simulink model "Requirements_Table"  (R2022b)
settings: Solver=FixedStepAuto  StartTime=0.0  StopTime=10.0  FixedStep=1e-3  RelTol=1e-3  EnableMultiTasking=on
undefined symbols (not defined in the file): D0, D1, D10, D11, D12, D13, D2, D3, D4, D5, D6, D7, D8, D9, PTA0, PTA1, PTA2, PTB23, PTB9, PTC16, PTC17, PTC2, PTC3, PTC4, PTD0, PTD1, PTD2, PTD3
libraries: frdmk64flib x17
settings Model: ExtModeTrigDuration=5  Creator=sarahalabdulrazzak  LastModifiedBy=shaydarahmatyan
settings SolverCC: AlgebraicLoopSolver=TrustRegion
settings OptimizationCC: EnhancedBackFolding=on  PassReuseOutputArgsAs=Individual arguments  ZeroExternalMemoryAtStartup=off  ZeroInternalMemoryAtStartup=off  MaxStackSize=64  OptimizeBlockOrder=speed  DifferentSizesBufferReuse=on  OptimizationCustomize=off  EfficientTunableParamExpr=on
settings DebuggingCC: ParameterTunabilityLossMsg=error  UnconnectedInputMsg=warning  UnconnectedOutputMsg=warning  UnconnectedLineMsg=warning  SFMachineParentedDataDiag=warning
settings HardwareCC: ProdBitPerPointer=32  ProdBitPerSizeT=32  ProdBitPerPtrDiffT=32  ProdLargestAtomicInteger=Long  ProdLargestAtomicFloat=Double  ProdWordSize=32  ProdHWDeviceType=ARM Compatible->ARM Cortex
settings ModelReferenceCC: EnableRefExpFcnMdlSchedulingChecks=on
settings SFSimCC: MATLABDynamicMemAlloc=off
settings RTWCC: Description=Embedded Coder  SystemTargetFile=ert.tlc  HardwareBoard=NXP FRDM-K64F  TLCOptions="-aInlineSetEventsForThisBaseRateFcn=TLC_FALSE -aSuppressMultiTaskScheduler=TLC_FALSE  -aRateBasedStepFcn=0"  TemplateMakefile=ert_default_tmf  Toolchain=GNU Tools for ARM Embedded Processors
settings CodeAppCC: ForceParamTrailComments=on  IgnoreCustomStorageClasses=off  OperatorAnnotations=on  SimulinkDataObjDesc=on  SFDataObjDesc=on  InsertBlockDesc=on

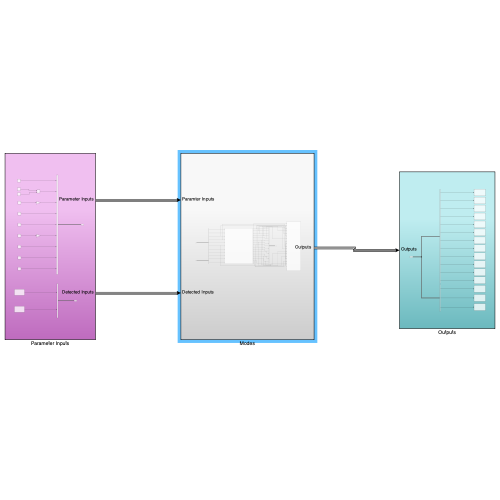
[thumbnail: Simulink's stored preview of the top-level diagram]
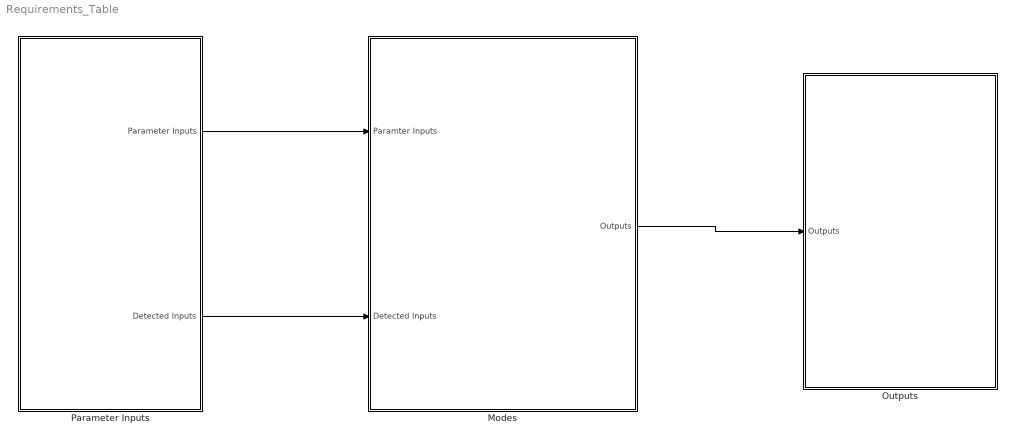
== system Requirements_Table ==
  Modes : Subsystem
  Outputs : Subsystem
  Parameter Inputs : Subsystem
  wires:
  Parameter Inputs/1(Parameter Inputs) -> Modes/1(Paramter Inputs)
  Parameter Inputs/2(Detected Inputs) -> Modes/2(Detected Inputs)
  Modes/1("Outputs ") -> Outputs/1("Outputs ")

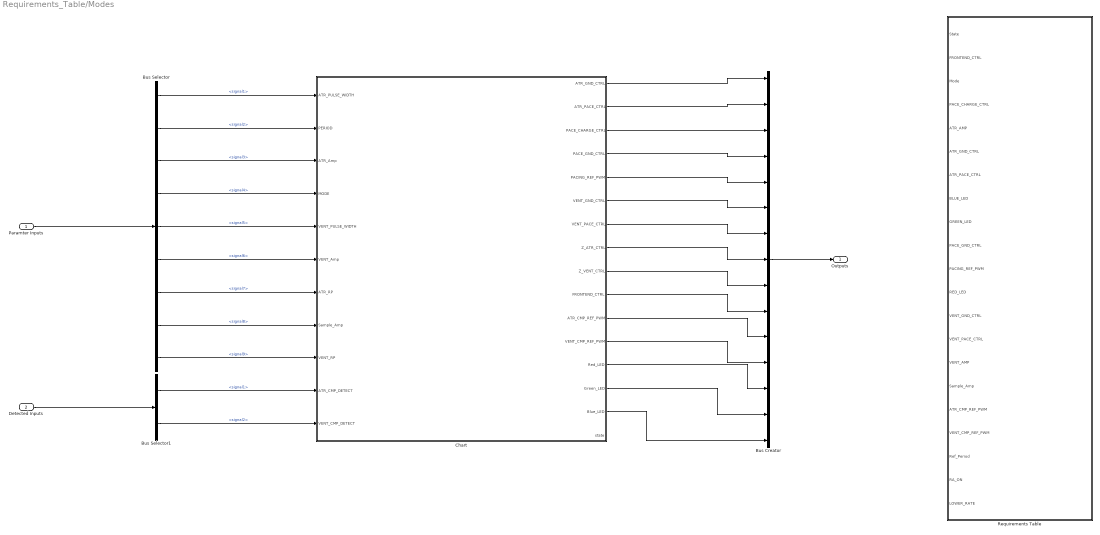
== system Requirements_Table/Modes ==
  Paramter Inputs : Inport
  Detected Inputs : Inport  Port=2
  Bus Creator : BusCreator  Inputs=15
  Bus Selector : BusSelector  OutputSignals=signal1,signal2,signal3,signal4,signal5,signal6,signal7,signal8,signal9
  Bus Selector1 : BusSelector  OutputSignals=signal1,signal2
  Chart : Stateflow chart  TreatAsAtomicUnit=on
  Requirements Table : Requirements Table  TreatAsAtomicUnit=on
  "Outputs " : Outport
  wires:
  Paramter Inputs/1 -> Bus Selector/1
  Detected Inputs/1 -> Bus Selector1/1
  Bus Selector/4 -> Chart/4(MODE)  "<signal4>"
  Bus Selector/5 -> Chart/5(VENT_PULSE_WIDTH)  "<signal5>"
  Bus Selector/6 -> Chart/6(VENT_Amp)  "<signal6>"
  Bus Selector/7 -> Chart/7(ATR_RP)  "<signal7>"
  Bus Selector/8 -> Chart/8(Sample_Amp)  "<signal8>"
  Bus Selector/9 -> Chart/9(VENT_RP)  "<signal9>"
  Bus Selector/1 -> Chart/1(ATR_PULSE_WIDTH)  "<signal1>"
  Bus Selector/2 -> Chart/2(PERIOD)  "<signal2>"
  Bus Selector/3 -> Chart/3(ATR_Amp)  "<signal3>"
  Chart/1(ATR_GND_CTRL) -> Bus Creator/1
  Chart/2(ATR_PACE_CTRL) -> Bus Creator/2
  Chart/4(PACE_GND_CTRL) -> Bus Creator/4
  Chart/5(PACING_REF_PWM) -> Bus Creator/5
  Chart/6(VENT_GND_CTRL) -> Bus Creator/6
  Chart/7(VENT_PACE_CTRL) -> Bus Creator/7
  Chart/8(Z_ATR_CTRL) -> Bus Creator/8
  Chart/9(Z_VENT_CTRL) -> Bus Creator/9
  Chart/10(FRONTEND_CTRL) -> Bus Creator/10
  Chart/11(ATR_CMP_REF_PWM) -> Bus Creator/11
  Chart/12(VENT_CMP_REF_PWM) -> Bus Creator/12
  Bus Creator/1 -> "Outputs "/1
  Chart/14(Green_LED) -> Bus Creator/14
  Chart/15(Blue_LED) -> Bus Creator/15
  Bus Selector1/1 -> Chart/10(ATR_CMP_DETECT)  "<signal1>"
  Bus Selector1/2 -> Chart/11(VENT_CMP_DETECT)  "<signal2>"
  Chart/3(PACE_CHARGE_CTRL) -> Bus Creator/3
  Chart/13(Red_LED) -> Bus Creator/13

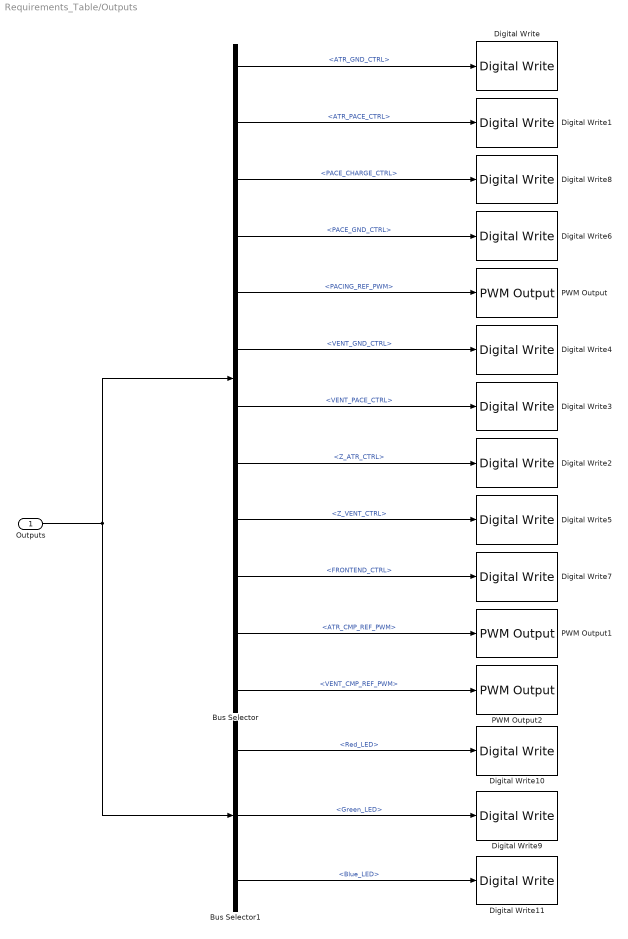
== system Requirements_Table/Outputs ==
  "Outputs " : Inport
  Bus Selector : BusSelector  OutputSignals=ATR_GND_CTRL,ATR_PACE_CTRL,PACE_CHARGE_CTRL,PACE_GND_CTRL,PACING_REF_PWM,VENT_GND_CTRL,VENT_PACE_CTRL,Z_ATR_CTRL,Z_VENT_CTRL,FRONTEND_CTRL,ATR_CMP_REF_PWM,VENT_CMP_REF_PWM
  Bus Selector1 : BusSelector  OutputSignals=Red_LED,Green_LED,Blue_LED
  Digital Write : frdmk64flib/Digital Write  Whichpin=PTD2 (D11)
  Digital Write1 : frdmk64flib/Digital Write  Whichpin=PTA0 (D8)
  Digital Write10 : frdmk64flib/Digital Write  Whichpin=RED_LED
  Digital Write11 : frdmk64flib/Digital Write  Whichpin=BLUE_LED
  Digital Write2 : frdmk64flib/Digital Write  Whichpin=PTB23 (D4)
  Digital Write3 : frdmk64flib/Digital Write  Whichpin=PTC4 (D9)
  Digital Write4 : frdmk64flib/Digital Write  Whichpin=PTD3 (D12)
  Digital Write5 : frdmk64flib/Digital Write  Whichpin=PTC3 (D7)
  Digital Write6 : frdmk64flib/Digital Write  Whichpin=PTD0 (D10)
  Digital Write7 : frdmk64flib/Digital Write  Whichpin=PTD1 (D13)
  Digital Write8 : frdmk64flib/Digital Write  Whichpin=PTB9 (D2)
  Digital Write9 : frdmk64flib/Digital Write  Whichpin=GREEN_LED
  PWM Output : frdmk64flib/PWM Output  Whichpin=PTA2 (D5)  InitialFrequency=2000  InitialDutyCycle=0
  PWM Output1 : frdmk64flib/PWM Output  Whichpin=PTC2 (D6)  InitialFrequency=2000  InitialDutyCycle=0
  PWM Output2 : frdmk64flib/PWM Output  Whichpin=PTA1 (D3)  InitialFrequency=2000  InitialDutyCycle=0
  wires:
  Bus Selector/1 -> Digital Write/1  "<ATR_GND_CTRL>"
  Bus Selector/2 -> Digital Write1/1  "<ATR_PACE_CTRL>"
  Bus Selector/3 -> Digital Write8/1  "<PACE_CHARGE_CTRL>"
  Bus Selector/4 -> Digital Write6/1  "<PACE_GND_CTRL>"
  Bus Selector/5 -> PWM Output/1  "<PACING_REF_PWM>"
  Bus Selector/6 -> Digital Write4/1  "<VENT_GND_CTRL>"
  Bus Selector/7 -> Digital Write3/1  "<VENT_PACE_CTRL>"
  Bus Selector/8 -> Digital Write2/1  "<Z_ATR_CTRL>"
  Bus Selector/9 -> Digital Write5/1  "<Z_VENT_CTRL>"
  Bus Selector/10 -> Digital Write7/1  "<FRONTEND_CTRL>"
  Bus Selector/11 -> PWM Output1/1  "<ATR_CMP_REF_PWM>"
  Bus Selector/12 -> PWM Output2/1  "<VENT_CMP_REF_PWM>"
  "Outputs "/1 -> Bus Selector/1, Bus Selector1/1
  Bus Selector1/1 -> Digital Write10/1  "<Red_LED>"
  Bus Selector1/2 -> Digital Write9/1  "<Green_LED>"
  Bus Selector1/3 -> Digital Write11/1  "<Blue_LED>"

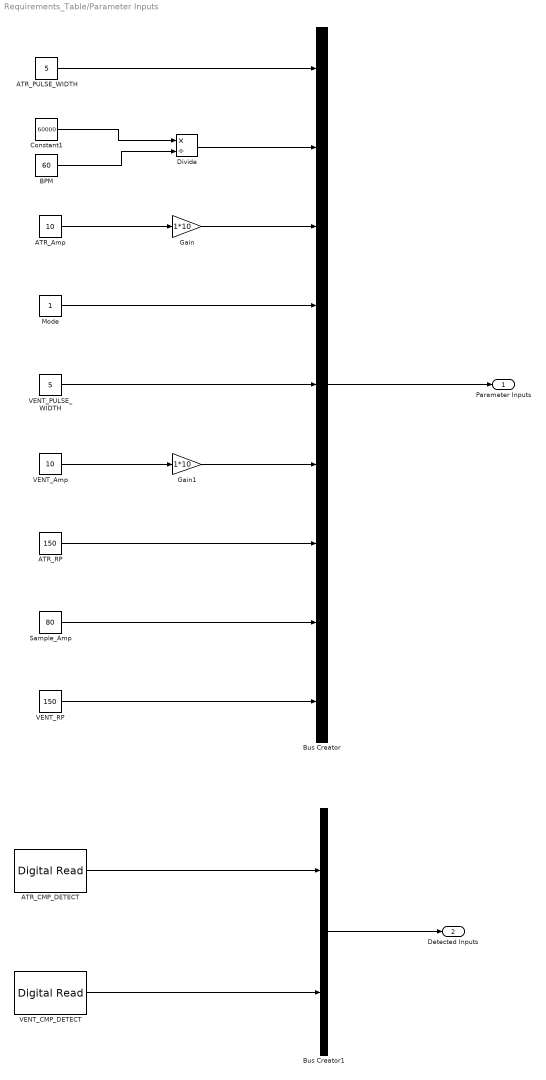
== system Requirements_Table/Parameter Inputs ==
  ATR_Amp : Constant  Value=10
  ATR_CMP_DETECT : frdmk64flib/Digital Read  Whichpin=PTC16 (D0)  SampleTime=-1
  ATR_PULSE_WIDTH : Constant  Value=5
  ATR_RP : Constant  Value=150
  BPM : Constant  Value=60
  Bus Creator : BusCreator  Inputs=9
  Bus Creator1 : BusCreator  Inputs=2
  Constant1 : Constant  Value=60000
  Divide : Product  Inputs=*/
  Gain : Gain  Gain=1*10
  Gain1 : Gain  Gain=1*10
  Mode : Constant
  Sample_Amp : Constant  Value=80
  VENT_Amp : Constant  Value=10
  VENT_CMP_DETECT : frdmk64flib/Digital Read  Whichpin=PTC17 (D1)  SampleTime=-1
  VENT_PULSE_WIDTH : Constant  Value=5
  VENT_RP : Constant  Value=150
  Parameter Inputs : Outport
  Detected Inputs : Outport  Port=2
  wires:
  Bus Creator/1 -> Parameter Inputs/1
  ATR_PULSE_WIDTH/1 -> Bus Creator/1
  BPM/1 -> Divide/2
  Constant1/1 -> Divide/1
  Divide/1 -> Bus Creator/2
  ATR_Amp/1 -> Gain/1
  Gain/1 -> Bus Creator/3
  Mode/1 -> Bus Creator/4
  VENT_PULSE_WIDTH/1 -> Bus Creator/5
  VENT_Amp/1 -> Gain1/1
  Gain1/1 -> Bus Creator/6
  ATR_RP/1 -> Bus Creator/7
  Sample_Amp/1 -> Bus Creator/8
  VENT_RP/1 -> Bus Creator/9
  Bus Creator1/1 -> Detected Inputs/1
  VENT_CMP_DETECT/1 -> Bus Creator1/2
  ATR_CMP_DETECT/1 -> Bus Creator1/1

== stateflow chart Requirements_Table/Modes/Requirements Table ==
  (default) -> (junction 1073743880)
  (junction 1073743880) -> (junction 1073743881) : {
      | % SF_REQ_REV_07
      | }
  (junction 1073743881) -> (junction 1073743883) : {
      | % HEADER_ASSIGNMENTS
      |
      | }
  (junction 1073743883) -> (junction 1073743885) : {
      | % START_A_4
      | }
  (junction 1073743885) -> (junction 1073743887) : {
      | }
  (junction 1073743887) -> (junction 1073743889) : {
      | reqtable_assumption(([0,3]), 4);
      | }
  (junction 1073743889) -> (junction 1073743891) : {
      | }
  (junction 1073743891) -> (junction 1073743893) : {
      | % END_A_4
      | }
  (junction 1073743893) -> (junction 1073743895) : {
      | % START_A_28
      | }
  (junction 1073743895) -> (junction 1073743897) : {
      | }
  (junction 1073743897) -> (junction 1073743899) : {
      | reqtable_assumption(([0,1]), 28);
      | }
  (junction 1073743899) -> (junction 1073743901) : {
      | }
  (junction 1073743901) -> (junction 1073743903) : {
      | % END_A_28
      | }
  (junction 1073743903) -> (junction 1073744078) : {
      | % START_R_1
      | }
  (junction 1073744078) -> (junction 1073744080) : {
      | }
  (junction 1073744080) -> (junction 1073744082)
  (junction 1073744082) -> (junction 1073744084) [order 1] : [(((Mode) == (1))) && (((State) == (0)))]
  (junction 1073744082) -> (junction 1073744100) [order 2]
  (junction 1073744084) -> (junction 1073744086) : {
      | reqtable_postcondition((((PACE_CHARGE_CTRL) == (1))) && (ATR_PACE_CTRL == 0) && (((PACING_REF_PWM ) == (ATR_AMP))) && (((PACE_CHARGE_CTRL) == (1))) && (((PACE_GND_CTRL) == (1))) && (ATR_GND_CTRL == 1) && (((RED_LED) == (0))) && (((GREEN_LED) == (0))) && (((BLUE_LED) == (0))) && (abs(time-get_param('SimulationTime')) / (60*1000) < LOWER_RATE), 'R:1');
      |
      | }
  (junction 1073744086) -> (junction 1073744088) : {
      | }
  (junction 1073744088) -> (junction 1073744577) : {
      | % START_R_34
      | }
  (junction 1073744577) -> (junction 1073744579) : {
      | }
  (junction 1073744579) -> (junction 1073744581)
  (junction 1073744581) -> (junction 1073744583) [order 1] : [(((RA_ON) == (0)))]
  (junction 1073744581) -> (junction 1073744589) [order 2]
  (junction 1073744583) -> (junction 1073744585)
  (junction 1073744585) -> (junction 1073744587) : {
      | }
  (junction 1073744587) -> (junction 1073744589)
  (junction 1073744589) -> (junction 1073744591)
  (junction 1073744591) -> (junction 1073744593) : {
      | % END_R_34
      | }
  (junction 1073744593) -> (junction 1073744661) : {
      | % START_R_37
      | }
  (junction 1073744661) -> (junction 1073744663) : {
      | }
  (junction 1073744663) -> (junction 1073744665)
  (junction 1073744665) -> (junction 1073744667) [order 1] : [(((RA_ON) == (1)))]
  (junction 1073744665) -> (junction 1073744673) [order 2]
  (junction 1073744667) -> (junction 1073744669)
  (junction 1073744669) -> (junction 1073744671) : {
      | }
  (junction 1073744671) -> (junction 1073744673)
  (junction 1073744673) -> (junction 1073744675)
  (junction 1073744675) -> (junction 1073744677) : {
      | % END_R_37
      | }
  (junction 1073744677) -> (junction 1073744100)
  (junction 1073744100) -> (junction 1073744102)
  (junction 1073744102) -> (junction 1073744104) : {
      | % END_R_1
      | }
  (junction 1073744104) -> (junction 1073744155) : {
      | % START_R_7
      | }
  (junction 1073744155) -> (junction 1073744157) : {
      | }
  (junction 1073744157) -> (junction 1073744159)
  (junction 1073744159) -> (junction 1073744161) [order 1] : [(((Mode) == (1))) && (((State) == (1)))]
  (junction 1073744159) -> (junction 1073744177) [order 2]
  (junction 1073744161) -> (junction 1073744163) : {
      | reqtable_postcondition((((PACE_CHARGE_CTRL) == (0))) && (ATR_PACE_CTRL == 1) && (((PACING_REF_PWM ) == (ATR_AMP))) && (((PACE_CHARGE_CTRL) == (0))) && (((PACE_GND_CTRL) == (1))) && (ATR_GND_CTRL == 0) && (((RED_LED) == (1))) && (((GREEN_LED) == (0))) && (((BLUE_LED) == (0))) && (abs(time-get_param('SimulationTime')) / (60*1000)  < LOWER_RATE), 'R:2');
      |
      | }
  (junction 1073744163) -> (junction 1073744165) : {
      | }
  (junction 1073744165) -> (junction 1073744598) : {
      | % START_R_40
      | }
  (junction 1073744598) -> (junction 1073744600) : {
      | }
  (junction 1073744600) -> (junction 1073744602)
  (junction 1073744602) -> (junction 1073744604) [order 1] : [(((RA_ON) == (0)))]
  (junction 1073744602) -> (junction 1073744610) [order 2]
  (junction 1073744604) -> (junction 1073744606)
  (junction 1073744606) -> (junction 1073744608) : {
      | }
  (junction 1073744608) -> (junction 1073744610)
  (junction 1073744610) -> (junction 1073744612)
  (junction 1073744612) -> (junction 1073744614) : {
      | % END_R_40
      | }
  (junction 1073744614) -> (junction 1073744682) : {
      | % START_R_43
      | }
  (junction 1073744682) -> (junction 1073744684) : {
      | }
  (junction 1073744684) -> (junction 1073744686)
  (junction 1073744686) -> (junction 1073744688) [order 1] : [(((RA_ON) == (1)))]
  (junction 1073744686) -> (junction 1073744694) [order 2]
  (junction 1073744688) -> (junction 1073744690)
  (junction 1073744690) -> (junction 1073744692) : {
      | }
  (junction 1073744692) -> (junction 1073744694)
  (junction 1073744694) -> (junction 1073744696)
  (junction 1073744696) -> (junction 1073744698) : {
      | % END_R_43
      | }
  (junction 1073744698) -> (junction 1073744177)
  (junction 1073744177) -> (junction 1073744179)
  (junction 1073744179) -> (junction 1073744181) : {
      | % END_R_7
      | }
  (junction 1073744181) -> (junction 1073744198) : {
      | % START_R_10
      | }
  (junction 1073744198) -> (junction 1073744200) : {
      | }
  (junction 1073744200) -> (junction 1073744202)
  (junction 1073744202) -> (junction 1073744204) [order 1] : [(((Mode) == (3))) && (((State) == (0)))]
  (junction 1073744202) -> (junction 1073744220) [order 2]
  (junction 1073744204) -> (junction 1073744206) : {
      | reqtable_postcondition((((PACE_CHARGE_CTRL) == (1))) && (VENT_PACE_CTRL == 0) && (((PACING_REF_PWM ) == (VENT_AMP))) && (((PACE_CHARGE_CTRL) == (1))) && (((PACE_GND_CTRL) == (1))) && (VENT_GND_CTRL == 1) && (((RED_LED) == (0))) && (((GREEN_LED) == (0))) && (((BLUE_LED) == (0))) && (abs(time-get_param('SimulationTime')) / (60*1000)  < LOWER_RATE), 'R:3');
      |
      | }
  (junction 1073744206) -> (junction 1073744208) : {
      | }
  (junction 1073744208) -> (junction 1073744640) : {
      | % START_R_46
      | }
  (junction 1073744640) -> (junction 1073744642) : {
      | }
  (junction 1073744642) -> (junction 1073744644)
  (junction 1073744644) -> (junction 1073744646) [order 1] : [(((RA_ON) == (0)))]
  (junction 1073744644) -> (junction 1073744652) [order 2]
  (junction 1073744646) -> (junction 1073744648)
  (junction 1073744648) -> (junction 1073744650) : {
      | }
  (junction 1073744650) -> (junction 1073744652)
  (junction 1073744652) -> (junction 1073744654)
  (junction 1073744654) -> (junction 1073744656) : {
      | % END_R_46
      | }
  (junction 1073744656) -> (junction 1073744703) : {
      | % START_R_49
      | }
  (junction 1073744703) -> (junction 1073744705) : {
      | }
  (junction 1073744705) -> (junction 1073744707)
  (junction 1073744707) -> (junction 1073744709) [order 1] : [(((RA_ON) == (1)))]
  (junction 1073744707) -> (junction 1073744715) [order 2]
  (junction 1073744709) -> (junction 1073744711)
  (junction 1073744711) -> (junction 1073744713) : {
      | }
  (junction 1073744713) -> (junction 1073744715)
  (junction 1073744715) -> (junction 1073744717)
  (junction 1073744717) -> (junction 1073744719) : {
      | % END_R_49
      | }
  (junction 1073744719) -> (junction 1073744220)
  (junction 1073744220) -> (junction 1073744222)
  (junction 1073744222) -> (junction 1073744224) : {
      | % END_R_10
      | }
  (junction 1073744224) -> (junction 1073744253) : {
      | % START_R_13
      | }
  (junction 1073744253) -> (junction 1073744255) : {
      | }
  (junction 1073744255) -> (junction 1073744257)
  (junction 1073744257) -> (junction 1073744259) [order 1] : [(((Mode) == (3))) && (((State) == (1)))]
  (junction 1073744257) -> (junction 1073744275) [order 2]
  (junction 1073744259) -> (junction 1073744261) : {
      | reqtable_postcondition((((PACE_CHARGE_CTRL) == (0))) && (VENT_PACE_CTRL == 1) && (((PACING_REF_PWM ) == (VENT_AMP))) && (((PACE_CHARGE_CTRL) == (0))) && (((PACE_GND_CTRL) == (1))) && (VENT_GND_CTRL == 0) && (((RED_LED) == (0))) && (((GREEN_LED) == (1))) && (((BLUE_LED) == (0))) && (abs(time-get_param('SimulationTime')) / (60*1000)  < LOWER_RATE), 'R:4');
      |
      | }
  (junction 1073744261) -> (junction 1073744263) : {
      | }
  (junction 1073744263) -> (junction 1073744619) : {
      | % START_R_52
      | }
  (junction 1073744619) -> (junction 1073744621) : {
      | }
  (junction 1073744621) -> (junction 1073744623)
  (junction 1073744623) -> (junction 1073744625) [order 1] : [(((RA_ON) == (0)))]
  (junction 1073744623) -> (junction 1073744631) [order 2]
  (junction 1073744625) -> (junction 1073744627)
  (junction 1073744627) -> (junction 1073744629) : {
      | }
  (junction 1073744629) -> (junction 1073744631)
  (junction 1073744631) -> (junction 1073744633)
  (junction 1073744633) -> (junction 1073744635) : {
      | % END_R_52
      | }
  (junction 1073744635) -> (junction 1073744724) : {
      | % START_R_55
      | }
  (junction 1073744724) -> (junction 1073744726) : {
      | }
  (junction 1073744726) -> (junction 1073744728)
  (junction 1073744728) -> (junction 1073744730) [order 1] : [(((RA_ON) == (1)))]
  (junction 1073744728) -> (junction 1073744736) [order 2]
  (junction 1073744730) -> (junction 1073744732)
  (junction 1073744732) -> (junction 1073744734) : {
      | }
  (junction 1073744734) -> (junction 1073744736)
  (junction 1073744736) -> (junction 1073744738)
  (junction 1073744738) -> (junction 1073744740) : {
      | % END_R_55
      | }
  (junction 1073744740) -> (junction 1073744275)
  (junction 1073744275) -> (junction 1073744277)
  (junction 1073744277) -> (junction 1073744279) : {
      | % END_R_13
      | }
  (junction 1073744279) -> (junction 1073744296) : {
      | % START_R_16
      | }
  (junction 1073744296) -> (junction 1073744298) : {
      | }
  (junction 1073744298) -> (junction 1073744300)
  (junction 1073744300) -> (junction 1073744302) [order 1] : [(((Mode) == (2))) && (((State) == (0))) && (FRONTEND_CTRL == 1) && (Ref_Period >100)]
  (junction 1073744300) -> (junction 1073744318) [order 2]
  (junction 1073744302) -> (junction 1073744304) : {
      | reqtable_postcondition((((PACE_CHARGE_CTRL) == (1))) && (ATR_PACE_CTRL == 0) && (((PACING_REF_PWM ) == (ATR_AMP))) && (((PACE_CHARGE_CTRL) == (1))) && (((PACE_GND_CTRL) == (1))) && (ATR_GND_CTRL == 1) && (((RED_LED) == (0))) && (((GREEN_LED) == (0))) && (((BLUE_LED) == (0))) && (ATR_CMP_REF_PWM == Sample_Amp) && (abs(time-get_param('SimulationTime')) / (60*1000)  < LOWER_RATE), 'R:5');
      |
      | }
  (junction 1073744304) -> (junction 1073744306) : {
      | }
  (junction 1073744306) -> (junction 1073744871) : {
      | % START_R_58
      | }
  (junction 1073744871) -> (junction 1073744873) : {
      | }
  (junction 1073744873) -> (junction 1073744875)
  (junction 1073744875) -> (junction 1073744877) [order 1] : [(((RA_ON) == (0)))]
  (junction 1073744875) -> (junction 1073744883) [order 2]
  (junction 1073744877) -> (junction 1073744879)
  (junction 1073744879) -> (junction 1073744881) : {
      | }
  (junction 1073744881) -> (junction 1073744883)
  (junction 1073744883) -> (junction 1073744885)
  (junction 1073744885) -> (junction 1073744887) : {
      | % END_R_58
      | }
  (junction 1073744887) -> (junction 1073744892) : {
      | % START_R_61
      | }
  (junction 1073744892) -> (junction 1073744894) : {
      | }
  (junction 1073744894) -> (junction 1073744896)
  (junction 1073744896) -> (junction 1073744898) [order 1] : [(((RA_ON) == (1)))]
  (junction 1073744896) -> (junction 1073744904) [order 2]
  (junction 1073744898) -> (junction 1073744900)
  (junction 1073744900) -> (junction 1073744902) : {
      | }
  (junction 1073744902) -> (junction 1073744904)
  (junction 1073744904) -> (junction 1073744906)
  (junction 1073744906) -> (junction 1073744908) : {
      | % END_R_61
      | }
  (junction 1073744908) -> (junction 1073744318)
  (junction 1073744318) -> (junction 1073744320)
  (junction 1073744320) -> (junction 1073744322) : {
      | % END_R_16
      | }
  (junction 1073744322) -> (junction 1073744373) : {
      | % START_R_19
      | }
  (junction 1073744373) -> (junction 1073744375) : {
      | }
  (junction 1073744375) -> (junction 1073744377)
  (junction 1073744377) -> (junction 1073744379) [order 1] : [(((Mode) == (2))) && (((State) == (1)))]
  (junction 1073744377) -> (junction 1073744395) [order 2]
  (junction 1073744379) -> (junction 1073744381) : {
      | reqtable_postcondition((((PACE_CHARGE_CTRL) == (0))) && (ATR_PACE_CTRL == 1) && (((PACING_REF_PWM ) == (ATR_AMP))) && (((PACE_CHARGE_CTRL) == (0))) && (((PACE_GND_CTRL) == (1))) && (ATR_GND_CTRL == 0) && (((RED_LED) == (0))) && (((GREEN_LED) == (0))) && (((BLUE_LED) == (0))) && (ATR_CMP_REF_PWM == Sample_Amp) && (abs(time-get_param('SimulationTime')) / (60*1000)  < LOWER_RATE), 'R:6');
      |
      | }
  (junction 1073744381) -> (junction 1073744383) : {
      | }
  (junction 1073744383) -> (junction 1073744745) : {
      | % START_R_64
      | }
  (junction 1073744745) -> (junction 1073744747) : {
      | }
  (junction 1073744747) -> (junction 1073744749)
  (junction 1073744749) -> (junction 1073744751) [order 1] : [(((RA_ON) == (0)))]
  (junction 1073744749) -> (junction 1073744757) [order 2]
  (junction 1073744751) -> (junction 1073744753)
  (junction 1073744753) -> (junction 1073744755) : {
      | }
  (junction 1073744755) -> (junction 1073744757)
  (junction 1073744757) -> (junction 1073744759)
  (junction 1073744759) -> (junction 1073744761) : {
      | % END_R_64
      | }
  (junction 1073744761) -> (junction 1073744766) : {
      | % START_R_67
      | }
  (junction 1073744766) -> (junction 1073744768) : {
      | }
  (junction 1073744768) -> (junction 1073744770)
  (junction 1073744770) -> (junction 1073744772) [order 1] : [(((RA_ON) == (1)))]
  (junction 1073744770) -> (junction 1073744778) [order 2]
  (junction 1073744772) -> (junction 1073744774)
  (junction 1073744774) -> (junction 1073744776) : {
      | }
  (junction 1073744776) -> (junction 1073744778)
  (junction 1073744778) -> (junction 1073744780)
  (junction 1073744780) -> (junction 1073744782) : {
      | % END_R_67
      | }
  (junction 1073744782) -> (junction 1073744395)
  (junction 1073744395) -> (junction 1073744397)
  (junction 1073744397) -> (junction 1073744399) : {
      | % END_R_19
      | }
  (junction 1073744399) -> (junction 1073744416) : {
      | % START_R_22
      | }
  (junction 1073744416) -> (junction 1073744418) : {
      | }
  (junction 1073744418) -> (junction 1073744420)
  (junction 1073744420) -> (junction 1073744422) [order 1] : [(((Mode) == (4))) && (((State) == (0))) && (FRONTEND_CTRL == 1) && (Ref_Period >100)]
  (junction 1073744420) -> (junction 1073744438) [order 2]
  (junction 1073744422) -> (junction 1073744424) : {
      | reqtable_postcondition((((PACE_CHARGE_CTRL) == (1))) && (VENT_PACE_CTRL == 0) && (((PACING_REF_PWM ) == (VENT_AMP))) && (((PACE_CHARGE_CTRL) == (1))) && (((PACE_GND_CTRL) == (1))) && (VENT_GND_CTRL == 1) && (((RED_LED) == (0))) && (((GREEN_LED) == (0))) && (((BLUE_LED) == (0))) && (VENT_CMP_REF_PWM == Sample_Amp) && (abs(time-get_param('SimulationTime')) / (60*1000)  < LOWER_RATE), 'R:7');
      |
      | }
  (junction 1073744424) -> (junction 1073744426) : {
      | }
  (junction 1073744426) -> (junction 1073744787) : {
      | % START_R_70
      | }
  (junction 1073744787) -> (junction 1073744789) : {
      | }
  (junction 1073744789) -> (junction 1073744791)
  (junction 1073744791) -> (junction 1073744793) [order 1] : [(((RA_ON) == (0)))]
  (junction 1073744791) -> (junction 1073744799) [order 2]
  (junction 1073744793) -> (junction 1073744795)
  (junction 1073744795) -> (junction 1073744797) : {
      | }
  (junction 1073744797) -> (junction 1073744799)
  (junction 1073744799) -> (junction 1073744801)
  (junction 1073744801) -> (junction 1073744803) : {
      | % END_R_70
      | }
  (junction 1073744803) -> (junction 1073744808) : {
      | % START_R_73
      | }
  (junction 1073744808) -> (junction 1073744810) : {
      | }
  (junction 1073744810) -> (junction 1073744812)
  (junction 1073744812) -> (junction 1073744814) [order 1] : [(((RA_ON) == (1)))]
  (junction 1073744812) -> (junction 1073744820) [order 2]
  (junction 1073744814) -> (junction 1073744816)
  (junction 1073744816) -> (junction 1073744818) : {
      | }
  (junction 1073744818) -> (junction 1073744820)
  (junction 1073744820) -> (junction 1073744822)
  (junction 1073744822) -> (junction 1073744824) : {
      | % END_R_73
      | }
  (junction 1073744824) -> (junction 1073744438)
  (junction 1073744438) -> (junction 1073744440)
  (junction 1073744440) -> (junction 1073744442) : {
      | % END_R_22
      | }
  (junction 1073744442) -> (junction 1073744493) : {
      | % START_R_25
      | }
  (junction 1073744493) -> (junction 1073744495) : {
      | }
  (junction 1073744495) -> (junction 1073744497)
  (junction 1073744497) -> (junction 1073744499) [order 1] : [(((Mode) == (4))) && (((State) == (1)))]
  (junction 1073744497) -> (junction 1073744515) [order 2]
  (junction 1073744499) -> (junction 1073744501) : {
      | reqtable_postcondition((((PACE_CHARGE_CTRL) == (0))) && (VENT_PACE_CTRL == 1) && (((PACING_REF_PWM ) == (VENT_AMP))) && (((PACE_CHARGE_CTRL) == (0))) && (((PACE_GND_CTRL) == (1))) && (VENT_GND_CTRL == 0) && (((RED_LED) == (0))) && (((GREEN_LED) == (1))) && (((BLUE_LED) == (0))) && (VENT_CMP_REF_PWM == Sample_Amp) && (abs(time-get_param('SimulationTime')) / (60*1000)  < LOWER_RATE), 'R:8');
      |
      | }
  (junction 1073744501) -> (junction 1073744503) : {
      | }
  (junction 1073744503) -> (junction 1073744829) : {
      | % START_R_76
      | }
  (junction 1073744829) -> (junction 1073744831) : {
      | }
  (junction 1073744831) -> (junction 1073744833)
  (junction 1073744833) -> (junction 1073744835) [order 1] : [(((RA_ON) == (0)))]
  (junction 1073744833) -> (junction 1073744841) [order 2]
  (junction 1073744835) -> (junction 1073744837)
  (junction 1073744837) -> (junction 1073744839) : {
      | }
  (junction 1073744839) -> (junction 1073744841)
  (junction 1073744841) -> (junction 1073744843)
  (junction 1073744843) -> (junction 1073744845) : {
      | % END_R_76
      | }
  (junction 1073744845) -> (junction 1073744850) : {
      | % START_R_79
      | }
  (junction 1073744850) -> (junction 1073744852) : {
      | }
  (junction 1073744852) -> (junction 1073744854)
  (junction 1073744854) -> (junction 1073744856) [order 1] : [(((RA_ON) == (1)))]
  (junction 1073744854) -> (junction 1073744862) [order 2]
  (junction 1073744856) -> (junction 1073744858)
  (junction 1073744858) -> (junction 1073744860) : {
      | }
  (junction 1073744860) -> (junction 1073744862)
  (junction 1073744862) -> (junction 1073744864)
  (junction 1073744864) -> (junction 1073744866) : {
      | % END_R_79
      | }
  (junction 1073744866) -> (junction 1073744515)
  (junction 1073744515) -> (junction 1073744517)
  (junction 1073744517) -> (junction 1073744519) : {
      | % END_R_25
      | }
  data: State input; FRONTEND_CTRL input; Mode input; PACE_CHARGE_CTRL input; ATR_AMP input; ATR_GND_CTRL input; ATR_PACE_CTRL input; BLUE_LED input; GREEN_LED input; PACE_GND_CTRL input; PACING_REF_PWM input; RED_LED input; VENT_GND_CTRL input; VENT_PACE_CTRL input; VENT_AMP input; Sample_Amp input; ATR_CMP_REF_PWM input; VENT_CMP_REF_PWM input; Ref_Period input; time local; RA_ON input; LOWER_RATE input

== stateflow chart Requirements_Table/Modes/Chart ==
  state AOO
    entry:
    state =0
    FRONTEND_CTRL = LOW
    %Charge primary capcitor C22
    ATR_PACE_CTRL=LOW
    VENT_PACE_CTRL=LOW
    PACING_REF_PWM = ATR_Amp
    PACE_CHARGE_CTRL = HIGH
    %Discharge block capacitor C21
    PACE_GND_CTRL = HIGH
    %VENT_PACE_CTRL = LOW
    Z_ATR_CTRL = LOW
    Z_VENT_CTRL = LOW
    %ATR_PACE_CTRL = LOW
    ATR_GND_CTRL = HIGH
    VENT_GND_CTRL = LOW
    %use LED  to verify state
    Red_LED=false
    Green_LED=false
    Blue_LED=false
  state Identify_Mode_Path
    entry:
    % MODE = 1 (AOO)
    % MODE = 2 (AAI)
    % MODE = 3 (VOO)
    % MODE = 4 (VVI)
    %
    %pacemaker disconnected
    %stop sensing
    PACE_CHARGE_CTRL = LOW
    VENT_PACE_CTRL = LOW
    ATR_PACE_CTRL = LOW
    PACE_GND_CTRL = LOW
    ATR_GND_CTRL = LOW
    VENT_GND_CTRL = LOW
    Z_ATR_CTRL = LOW
    Z_VENT_CTRL = LOW
    FRONTEND_CTRL = LOW
  state AOO_ATR_PULSE
    entry:
    state = 1
    FRONTEND_CTRL = LOW
    %Discharge C22 primary capacitor
    %Charge C21 block capacitor
    PACE_CHARGE_CTRL = LOW
    PACE_GND_CTRL = HIGH
    ATR_PACE_CTRL = HIGH
    ATR_GND_CTRL = LOW
    Z_ATR_CTRL = LOW
    Z_VENT_CTRL = LOW
    VENT_GND_CTRL = LOW
    VENT_PACE_CTRL  = LOW
    PACING_REF_PWM = ATR_Amp
    %use LED  to verify state
    Red_LED=true
    Green_LED=false
    Blue_LED=false
  state AAI
    entry:
    state =0
    %sensing ON
    FRONTEND_CTRL = HIGH
    %Charge primary capcitor C22
    ATR_PACE_CTRL=LOW
    VENT_PACE_CTRL=LOW
    PACING_REF_PWM = ATR_Amp
    PACE_CHARGE_CTRL = HIGH
    %Discharge block capacitor C21
    PACE_GND_CTRL = HIGH
    VENT_PACE_CTRL = LOW
    Z_ATR_CTRL = LOW
    Z_VENT_CTRL = LOW
    ATR_GND_CTRL = HIGH
    VENT_GND_CTRL = LOW
    ATR_CMP_REF_PWM = Sample_Amp
    %use LED  to verify state
    Red_LED=false
    Blue_LED=false
    Green_LED=false
  state AAI_ATR_PULSE
    state =1
    entry:
    %sensing OFF
    FRONTEND_CTRL = LOW
    %Discharge C22 primary capacitor
    %Charge C21 block capacitor
    PACE_CHARGE_CTRL = LOW
    PACE_GND_CTRL = HIGH
    ATR_PACE_CTRL = HIGH
    ATR_GND_CTRL = LOW
    Z_ATR_CTRL = LOW
    Z_VENT_CTRL = LOW
    VENT_GND_CTRL = LOW
    VENT_PACE_CTRL  = LOW
    PACING_REF_PWM = ATR_Amp
    %use LED  to verify state
    Red_LED=false
    Green_LED=false
    Blue_LED=true
  state VOO
    entry:
    state =0
    FRONTEND_CTRL = LOW
    %Charge primary capcitor C22
    ATR_PACE_CTRL=LOW
    VENT_PACE_CTRL=LOW
    PACING_REF_PWM = VENT_Amp
    PACE_CHARGE_CTRL = HIGH
    %Discharge block capacitor C21
    PACE_GND_CTRL = HIGH
    %VENT_PACE_CTRL = LOW
    Z_ATR_CTRL = LOW
    Z_VENT_CTRL = LOW
    %ATR_PACE_CTRL = LOW
    ATR_GND_CTRL = LOW
    VENT_GND_CTRL = HIGH
    %use LED  to verify state
    Red_LED=false
    Green_LED=false
    Blue_LED=false
  state VOO_VENT_PULSE
    entry:
    state =1
    FRONTEND_CTRL = LOW
    %Discharge C22 primary capacitor
    %Charge C21 block capacitor
    PACE_CHARGE_CTRL = LOW
    PACE_GND_CTRL = HIGH
    ATR_PACE_CTRL = LOW
    ATR_GND_CTRL = LOW
    Z_ATR_CTRL = LOW
    Z_VENT_CTRL = LOW
    VENT_GND_CTRL = LOW
    VENT_PACE_CTRL  = HIGH
    PACING_REF_PWM = VENT_Amp
    %use LED  to verify state
    Red_LED=false
    Green_LED=true
    Blue_LED=false
  state VVI
    entry:
    state = 0
    %sensing ON
    FRONTEND_CTRL = HIGH
    %Charge primary capcitor C22
    ATR_PACE_CTRL=LOW
    VENT_PACE_CTRL= LOW
    PACING_REF_PWM = VENT_Amp
    PACE_CHARGE_CTRL = HIGH
    %Discharge block capacitor C21
    PACE_GND_CTRL = HIGH
    VENT_PACE_CTRL = LOW
    Z_ATR_CTRL = LOW
    Z_VENT_CTRL = LOW
    ATR_GND_CTRL = LOW
    VENT_GND_CTRL = HIGH
    VENT_CMP_REF_PWM = Sample_Amp
    %use LED  to verify state
    Red_LED=true
    Green_LED=false
    Blue_LED=false
  state VVI_VENT_PULSE
    entry:
    state = 1
    %sensing OFF
    FRONTEND_CTRL = LOW
    %Discharge C22 primary capacitor
    %Charge C21 block capacitor
    PACE_CHARGE_CTRL = LOW
    PACE_GND_CTRL = HIGH
    ATR_PACE_CTRL = LOW
    ATR_GND_CTRL = LOW
    Z_ATR_CTRL = LOW
    Z_VENT_CTRL = LOW
    VENT_GND_CTRL = LOW
    VENT_PACE_CTRL  = HIGH
    PACING_REF_PWM = VENT_Amp
    %use LED  to verify state
    Red_LED=false
    Green_LED=true
    Blue_LED=false
  (default) -> Identify_Mode_Path
  AOO -> AOO_ATR_PULSE : after(PERIOD - ATR_PULSE_WIDTH,msec)
  Identify_Mode_Path -> AOO [order 1] : [MODE == 1]
  AOO_ATR_PULSE -> AOO : after(ATR_PULSE_WIDTH,msec)
  AAI_ATR_PULSE -> AAI : after(ATR_PULSE_WIDTH,msec)
  Identify_Mode_Path -> AAI [order 2] : [MODE == 2]
  AAI -> (junction 41)
  (junction 41) -> AAI_ATR_PULSE [order 1] : after(PERIOD - ATR_PULSE_WIDTH,msec)[ATR_CMP_DETECT == LOW]
  (junction 41) -> (junction 35) [order 2] : [ATR_CMP_DETECT == HIGH]
  (junction 35) -> AAI : after(ATR_RP, msec)
  VOO -> VOO_VENT_PULSE : after(PERIOD - VENT_PULSE_WIDTH,msec)
  Identify_Mode_Path -> VOO [order 3] : [MODE == 3]
  VOO_VENT_PULSE -> VOO : after(VENT_PULSE_WIDTH,msec)
  VVI_VENT_PULSE -> VVI : after(VENT_PULSE_WIDTH,msec)
  Identify_Mode_Path -> VVI [order 4] : [MODE == 4]
  VVI -> (junction 61)
  (junction 61) -> VVI_VENT_PULSE [order 1] : after(PERIOD - VENT_PULSE_WIDTH,msec)[VENT_CMP_DETECT == LOW]
  (junction 61) -> (junction 59) [order 2] : [VENT_CMP_DETECT == HIGH]
  (junction 59) -> VVI : after(VENT_RP, msec)
  data: ATR_PULSE_WIDTH input; PERIOD input; ATR_Amp input; MODE input; VENT_PULSE_WIDTH input; VENT_Amp input; ATR_RP input; Sample_Amp input; VENT_RP input; ATR_CMP_DETECT input; VENT_CMP_DETECT input; HIGH local =1; LOW local =0; ATR_GND_CTRL output; ATR_PACE_CTRL output; PACE_CHARGE_CTRL output; PACE_GND_CTRL output; PACING_REF_PWM output; VENT_GND_CTRL output; VENT_PACE_CTRL output; Z_ATR_CTRL output; Z_VENT_CTRL output; FRONTEND_CTRL output; ATR_CMP_REF_PWM output; VENT_CMP_REF_PWM output; Red_LED output; Green_LED output; Blue_LED output; state output
